simulink model "main_SIM_MMP_IIR"  (R2024a)
settings: Solver=VariableStepAuto  StartTime=0.0  StopTime=Tsim  FixedStep=simStepSize  RelTol=1e-3
undefined symbols (not defined in the file): A_amp, B_para, f_d, ForceDist, L_t, p_off, Ps_sys, Pz_sys, Qcvx_FIR, Qcvx_IIR, SensorNoise, Ts, Tu, w_k, w_k_IIR
libraries: cstblocks x4
settings Model: Creator=tomli  LastModifiedBy=tpjch
settings RTWCC: GPUComputeCapability=3.5

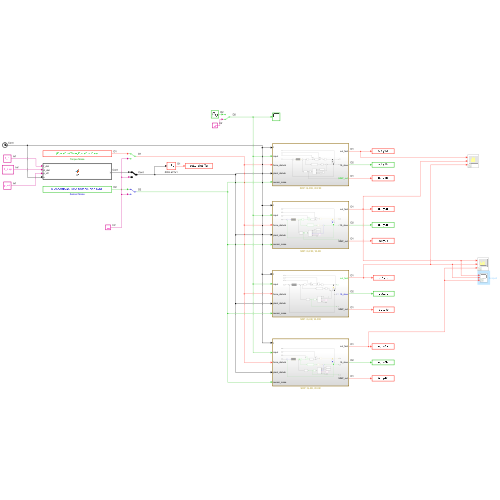
[thumbnail: Simulink's stored preview of the top-level diagram]
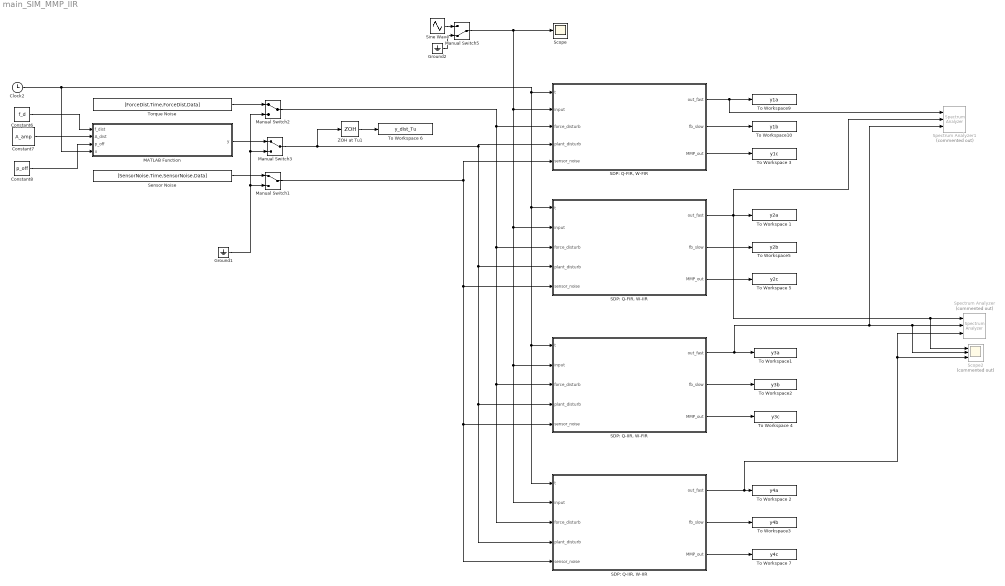
== system main_SIM_MMP_IIR ==
  Clock2 : Clock
  Constant6 : Constant  Value=f_d
  Constant7 : Constant  Value=A_amp
  Constant8 : Constant  Value=p_off
  Ground1 : Ground
  Ground2 : Ground
  MATLAB Function : MATLAB Function  TreatAsAtomicUnit=on
  Manual Switch1 : ManualSwitch
  Manual Switch2 : ManualSwitch
  Manual Switch3 : ManualSwitch
  Manual Switch5 : ManualSwitch  CurrentSetting=0
  "SDP: Q-FIR, W-FIR" : Subsystem
  "SDP: Q-FIR, W-IIR" : Subsystem
  "SDP: Q-IIR, W-FIR" : Subsystem
  "SDP: Q-IIR, W-IIR" : Subsystem
  Scope : Scope
  Scope2 : Scope  Commented=on  NumInputPorts=3
  Sensor Noise : FromWorkspace  VariableName=[SensorNoise.Time,SensorNoise.Data]  SampleTime=SensorNoise.Ts  Interpolate=off  ZeroCross=off  OutputAfterFinalValue=Setting to zero
  Sine Wave : Sin  SampleTime=Ts
  Spectrum Analyzer : SpectrumAnalyzer  Commented=on  NumInputPorts=3  WindowPosition=[1.000000,49.000000,1536.000000,888.000000,]  ScopeFrameLocation=window  Span=5280  StartFrequency=-2640  StopFrequency=2640  YLimits=[-62.09679226,16.22908912]  ShowLegend=on
  Spectrum Analyzer1 : SpectrumAnalyzer  Commented=on  NumInputPorts=3  WindowPosition=[1.000000,49.000000,1536.000000,888.000000,]  ScopeFrameLocation=window  Span=5280  StartFrequency=-2640  StopFrequency=2640  YLimits=[-59.07736824,14.75660534]  ShowLegend=on
  To Workspace 1 : ToWorkspace  VariableName=y2a  SaveFormat=Structure With Time  SampleTime=Tu
      settings: MaxDataPoints=Inf
  To Workspace 2 : ToWorkspace  VariableName=y4a  SaveFormat=Structure With Time  SampleTime=Tu
      settings: MaxDataPoints=Inf
  To Workspace 3 : ToWorkspace  VariableName=y1c  SaveFormat=Structure With Time  SampleTime=Tu
      settings: MaxDataPoints=Inf
  To Workspace 4 : ToWorkspace  VariableName=y3c  SaveFormat=Structure With Time  SampleTime=Tu
      settings: MaxDataPoints=Inf
  To Workspace 5 : ToWorkspace  VariableName=y2c  SaveFormat=Structure With Time  SampleTime=Tu
      settings: MaxDataPoints=Inf
  To Workspace 6 : ToWorkspace  VariableName=y_dist_Tu  SaveFormat=Structure With Time  SampleTime=Tu
      settings: MaxDataPoints=Inf
  To Workspace 7 : ToWorkspace  VariableName=y4c  SaveFormat=Structure With Time  SampleTime=Tu
      settings: MaxDataPoints=Inf
  To Workspace1 : ToWorkspace  VariableName=y3a  SaveFormat=Structure With Time  SampleTime=-1
  To Workspace10 : ToWorkspace  VariableName=y1b  SaveFormat=Structure With Time  SampleTime=-1
  To Workspace2 : ToWorkspace  VariableName=y3b  SaveFormat=Structure With Time  SampleTime=-1
  To Workspace3 : ToWorkspace  VariableName=y4b  SaveFormat=Structure With Time  SampleTime=Ts
  To Workspace5 : ToWorkspace  VariableName=y2b  SaveFormat=Structure With Time  SampleTime=Ts
  To Workspace9 : ToWorkspace  VariableName=y1a  SaveFormat=Structure With Time  SampleTime=-1
  Torque Noise : FromWorkspace  VariableName=[ForceDist.Time,ForceDist.Data]  SampleTime=ForceDist.Ts  Interpolate=off  ZeroCross=off  OutputAfterFinalValue=Setting to zero
  ZOH at Tu1 : ZeroOrderHold  SampleTime=Tu
  wires:
  Torque Noise/1 -> Manual Switch2/1
  Ground1/1 -> Manual Switch2/2, Manual Switch3/2, Manual Switch1/2
  Constant8/1 -> MATLAB Function/3(p_off)
  Constant7/1 -> MATLAB Function/2(A_dist)
  Constant6/1 -> MATLAB Function/1(f_dist)
  Sensor Noise/1 -> Manual Switch1/1
  MATLAB Function/1(y) -> Manual Switch3/1
  "SDP: Q-FIR, W-IIR"/3(MMP_out) -> To Workspace 5/1
  "SDP: Q-FIR, W-FIR"/1(out_fast) -> Spectrum Analyzer1/1, To Workspace9/1
  Sine Wave/1 -> Manual Switch5/1
  Ground2/1 -> Manual Switch5/2
  "SDP: Q-FIR, W-FIR"/2(fb_slow) -> To Workspace10/1
  "SDP: Q-FIR, W-IIR"/2(fb_slow) -> To Workspace5/1
  "SDP: Q-FIR, W-FIR"/3(MMP_out) -> To Workspace 3/1
  ZOH at Tu1/1 -> To Workspace 6/1
  "SDP: Q-IIR, W-FIR"/2(fb_slow) -> To Workspace2/1
  "SDP: Q-IIR, W-FIR"/3(MMP_out) -> To Workspace 4/1
  "SDP: Q-IIR, W-IIR"/2(fb_slow) -> To Workspace3/1
  "SDP: Q-IIR, W-FIR"/1(out_fast) -> Spectrum Analyzer1/3, Scope2/2, Spectrum Analyzer/2, To Workspace1/1
  Manual Switch5/1 -> "SDP: Q-IIR, W-IIR"/2(input), "SDP: Q-IIR, W-FIR"/2(input), "SDP: Q-FIR, W-IIR"/2(input), "SDP: Q-FIR, W-FIR"/2(input), Scope/1
  Manual Switch1/1 -> "SDP: Q-FIR, W-FIR"/5(sensor_noise), "SDP: Q-IIR, W-IIR"/5(sensor_noise), "SDP: Q-IIR, W-FIR"/5(sensor_noise), "SDP: Q-FIR, W-IIR"/5(sensor_noise)
  Manual Switch2/1 -> "SDP: Q-IIR, W-IIR"/3(force_disturb), "SDP: Q-IIR, W-FIR"/3(force_disturb), "SDP: Q-FIR, W-IIR"/3(force_disturb), "SDP: Q-FIR, W-FIR"/3(force_disturb)
  Clock2/1 -> "SDP: Q-IIR, W-IIR"/1(t), "SDP: Q-IIR, W-FIR"/1(t), "SDP: Q-FIR, W-IIR"/1(t), "SDP: Q-FIR, W-FIR"/1(t), MATLAB Function/4(u)
  Manual Switch3/1 -> ZOH at Tu1/1, "SDP: Q-IIR, W-IIR"/4(plant_disturb), "SDP: Q-IIR, W-FIR"/4(plant_disturb), "SDP: Q-FIR, W-IIR"/4(plant_disturb), "SDP: Q-FIR, W-FIR"/4(plant_disturb)
  "SDP: Q-IIR, W-IIR"/3(MMP_out) -> To Workspace 7/1
  "SDP: Q-IIR, W-IIR"/1(out_fast) -> Scope2/3, Spectrum Analyzer/3, To Workspace 2/1
  "SDP: Q-FIR, W-IIR"/1(out_fast) -> Spectrum Analyzer1/2, Scope2/1, Spectrum Analyzer/1, To Workspace 1/1

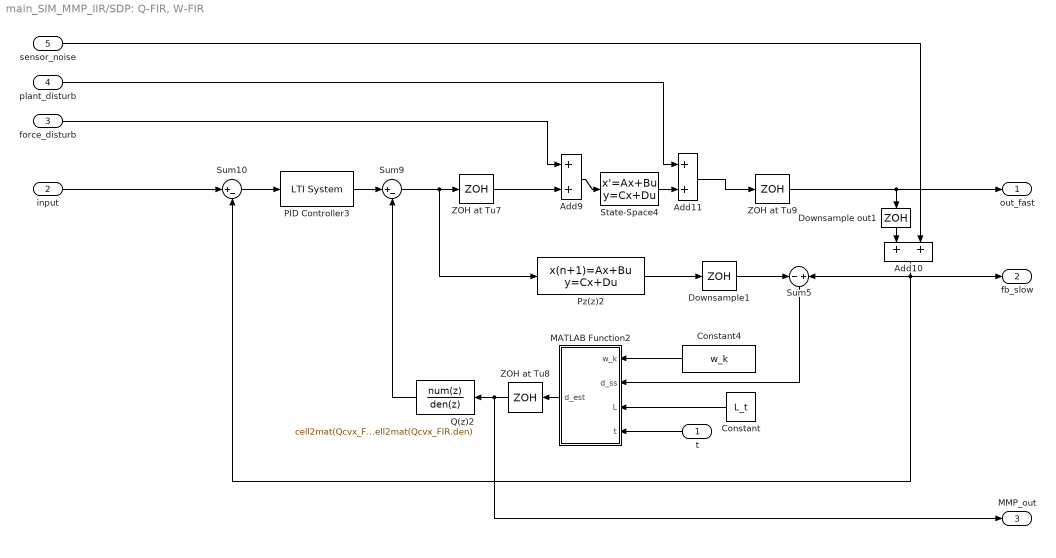
== system main_SIM_MMP_IIR/SDP: Q-FIR, W-FIR ==
  t : Inport
  input : Inport  Port=2
  force_disturb : Inport  Port=3
  plant_disturb : Inport  Port=4
  sensor_noise : Inport  Port=5
  Add10 : Sum
  Add11 : Sum
  Add9 : Sum
  Constant : Constant  Value=L_t
  Constant4 : Constant  Value=w_k
  Downsample out1 : ZeroOrderHold  SampleTime=Ts
  Downsample1 : ZeroOrderHold  SampleTime=Ts
  MATLAB Function2 : MATLAB Function  TreatAsAtomicUnit=on  SystemSampleTime=Tu
  PID Controller3 : cstblocks/LTI System  sys=Cz  IC=[]  PadeOrder=0
  Pz(z)2 : DiscreteStateSpace  A=Pz_sys.A  B=Pz_sys.B  C=Pz_sys.C  D=Pz_sys.D  SampleTime=Tu
  Q(z)2 : DiscreteTransferFcn  Numerator=cell2mat(Qcvx_FIR.num)  Denominator=cell2mat(Qcvx_FIR.den)  SampleTime=Tu
  State-Space4 : StateSpace  A=Ps_sys.A  B=Ps_sys.B  C=Ps_sys.C  D=Ps_sys.D  InitialCondition=0
  Sum10 : Sum  Inputs=|+-
  Sum5 : Sum  Inputs=-|+
  Sum9 : Sum  Inputs=|+-
  ZOH at Tu7 : ZeroOrderHold  SampleTime=Tu
  ZOH at Tu8 : ZeroOrderHold  SampleTime=Tu
  ZOH at Tu9 : ZeroOrderHold  SampleTime=Tu
  out_fast : Outport
  fb_slow : Outport  Port=2
  MMP_out : Outport  Port=3
  wires:
  ZOH at Tu9/1 -> Downsample out1/1, out_fast/1
  Sum9/1 -> Pz(z)2/1, ZOH at Tu7/1
  State-Space4/1 -> Add11/2
  Constant4/1 -> MATLAB Function2/1(w_k)
  Add10/1 -> Sum5/2, Sum10/2, fb_slow/1
  MATLAB Function2/1(d_est) -> ZOH at Tu8/1
  Add11/1 -> ZOH at Tu9/1
  force_disturb/1 -> Add9/1
  input/1 -> Sum10/1
  Pz(z)2/1 -> Downsample1/1
  ZOH at Tu8/1 -> MMP_out/1, Q(z)2/1
  Sum10/1 -> PID Controller3/1
  Add9/1 -> State-Space4/1
  Q(z)2/1 -> Sum9/2
  ZOH at Tu7/1 -> Add9/2
  Downsample1/1 -> Sum5/1
  Constant/1 -> MATLAB Function2/3(L)
  plant_disturb/1 -> Add11/1
  t/1 -> MATLAB Function2/4(t)
  sensor_noise/1 -> Add10/2
  Downsample out1/1 -> Add10/1
  Sum5/1 -> MATLAB Function2/2(d_ss)
  PID Controller3/1 -> Sum9/1

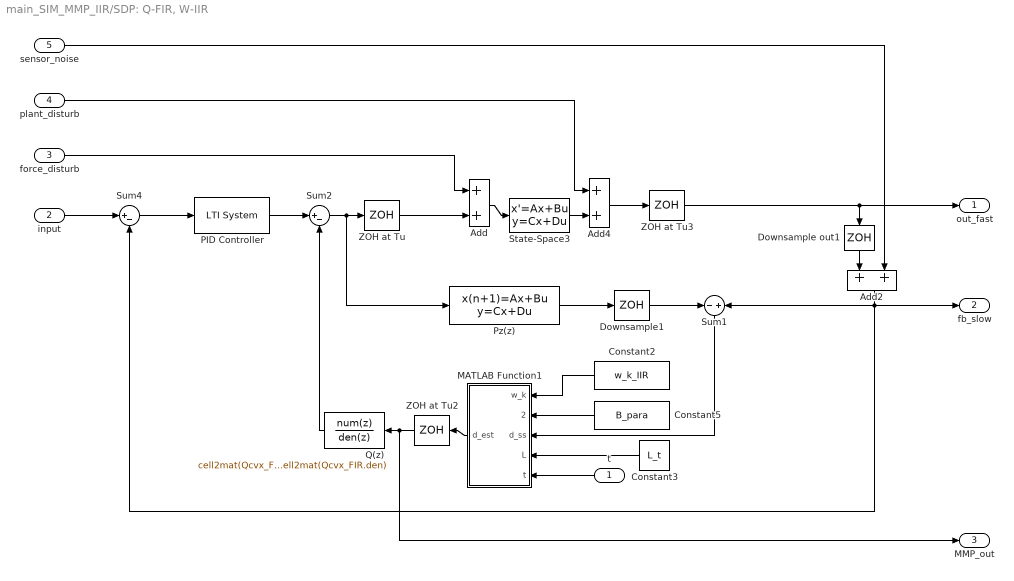
== system main_SIM_MMP_IIR/SDP: Q-FIR, W-IIR ==
  t : Inport
  input : Inport  Port=2
  force_disturb : Inport  Port=3
  plant_disturb : Inport  Port=4
  sensor_noise : Inport  Port=5
  Add : Sum
  Add2 : Sum
  Add4 : Sum
  Constant2 : Constant  Value=w_k_IIR
  Constant3 : Constant  Value=L_t
  Constant5 : Constant  Value=B_para
  Downsample out1 : ZeroOrderHold  SampleTime=Ts
  Downsample1 : ZeroOrderHold  SampleTime=Ts
  MATLAB Function1 : MATLAB Function  TreatAsAtomicUnit=on  SystemSampleTime=Tu
  PID Controller : cstblocks/LTI System  sys=Cz  IC=[]  PadeOrder=0
  Pz(z) : DiscreteStateSpace  A=Pz_sys.A  B=Pz_sys.B  C=Pz_sys.C  D=Pz_sys.D  SampleTime=Tu
  Q(z) : DiscreteTransferFcn  Numerator=cell2mat(Qcvx_FIR.num)  Denominator=cell2mat(Qcvx_FIR.den)  SampleTime=Tu
  State-Space3 : StateSpace  A=Ps_sys.A  B=Ps_sys.B  C=Ps_sys.C  D=Ps_sys.D  InitialCondition=0
  Sum1 : Sum  Inputs=-|+
  Sum2 : Sum  Inputs=|+-
  Sum4 : Sum  Inputs=|+-
  ZOH at Tu : ZeroOrderHold  SampleTime=Tu
  ZOH at Tu2 : ZeroOrderHold  SampleTime=Tu
  ZOH at Tu3 : ZeroOrderHold  SampleTime=Tu
  out_fast : Outport
  fb_slow : Outport  Port=2
  MMP_out : Outport  Port=3
  wires:
  Pz(z)/1 -> Downsample1/1
  ZOH at Tu/1 -> Add/2
  Add2/1 -> Sum1/2, Sum4/2, fb_slow/1
  Sum4/1 -> PID Controller/1
  State-Space3/1 -> Add4/2
  Downsample1/1 -> Sum1/1
  ZOH at Tu3/1 -> Downsample out1/1, out_fast/1
  Add4/1 -> ZOH at Tu3/1
  ZOH at Tu2/1 -> Q(z)/1, MMP_out/1
  Add/1 -> State-Space3/1
  Sum2/1 -> Pz(z)/1, ZOH at Tu/1
  Q(z)/1 -> Sum2/2
  force_disturb/1 -> Add/1
  plant_disturb/1 -> Add4/1
  sensor_noise/1 -> Add2/2
  input/1 -> Sum4/1
  Downsample out1/1 -> Add2/1
  Constant5/1 -> MATLAB Function1/2(B_para)
  Constant2/1 -> MATLAB Function1/1(w_k)
  MATLAB Function1/1(d_est) -> ZOH at Tu2/1
  Sum1/1 -> MATLAB Function1/3(d_ss)
  Constant3/1 -> MATLAB Function1/4(L)
  t/1 -> MATLAB Function1/5(t)
  PID Controller/1 -> Sum2/1

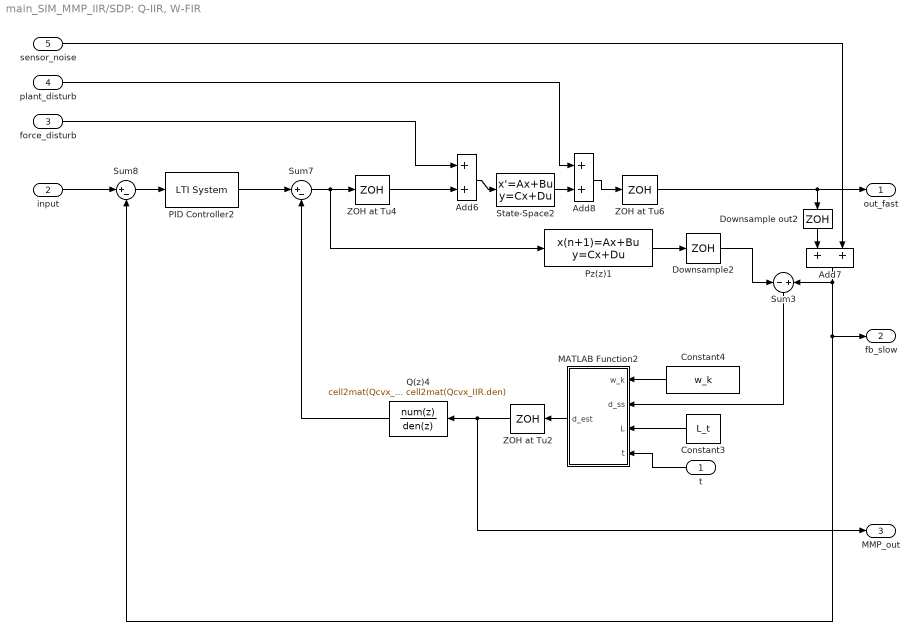
== system main_SIM_MMP_IIR/SDP: Q-IIR, W-FIR ==
  t : Inport
  input : Inport  Port=2
  force_disturb : Inport  Port=3
  plant_disturb : Inport  Port=4
  sensor_noise : Inport  Port=5
  Add6 : Sum
  Add7 : Sum
  Add8 : Sum
  Constant3 : Constant  Value=L_t
  Constant4 : Constant  Value=w_k
  Downsample out2 : ZeroOrderHold  SampleTime=Ts
  Downsample2 : ZeroOrderHold  SampleTime=Ts
  MATLAB Function2 : MATLAB Function  TreatAsAtomicUnit=on  SystemSampleTime=Tu
  PID Controller2 : cstblocks/LTI System  sys=Cz  IC=[]  PadeOrder=0
  Pz(z)1 : DiscreteStateSpace  A=Pz_sys.A  B=Pz_sys.B  C=Pz_sys.C  D=Pz_sys.D  SampleTime=Tu
  Q(z)4 : DiscreteTransferFcn  Numerator=cell2mat(Qcvx_IIR.num)  Denominator=cell2mat(Qcvx_IIR.den)
  State-Space2 : StateSpace  A=Ps_sys.A  B=Ps_sys.B  C=Ps_sys.C  D=Ps_sys.D  InitialCondition=0
  Sum3 : Sum  Inputs=-|+
  Sum7 : Sum  Inputs=|+-
  Sum8 : Sum  Inputs=|+-
  ZOH at Tu2 : ZeroOrderHold  SampleTime=Tu
  ZOH at Tu4 : ZeroOrderHold  SampleTime=Tu
  ZOH at Tu6 : ZeroOrderHold  SampleTime=Tu
  out_fast : Outport
  fb_slow : Outport  Port=2
  MMP_out : Outport  Port=3
  wires:
  Downsample2/1 -> Sum3/1
  Add8/1 -> ZOH at Tu6/1
  ZOH at Tu6/1 -> out_fast/1, Downsample out2/1
  ZOH at Tu4/1 -> Add6/2
  Add7/1 -> fb_slow/1, Sum8/2, Sum3/2
  input/1 -> Sum8/1
  sensor_noise/1 -> Add7/2
  Add6/1 -> State-Space2/1
  Sum8/1 -> PID Controller2/1
  State-Space2/1 -> Add8/2
  Sum7/1 -> Pz(z)1/1, ZOH at Tu4/1
  Pz(z)1/1 -> Downsample2/1
  plant_disturb/1 -> Add8/1
  force_disturb/1 -> Add6/1
  Downsample out2/1 -> Add7/1
  PID Controller2/1 -> Sum7/1
  Q(z)4/1 -> Sum7/2
  Constant3/1 -> MATLAB Function2/3(L)
  MATLAB Function2/1(d_est) -> ZOH at Tu2/1
  t/1 -> MATLAB Function2/4(t)
  Sum3/1 -> MATLAB Function2/2(d_ss)
  ZOH at Tu2/1 -> MMP_out/1, Q(z)4/1
  Constant4/1 -> MATLAB Function2/1(w_k)

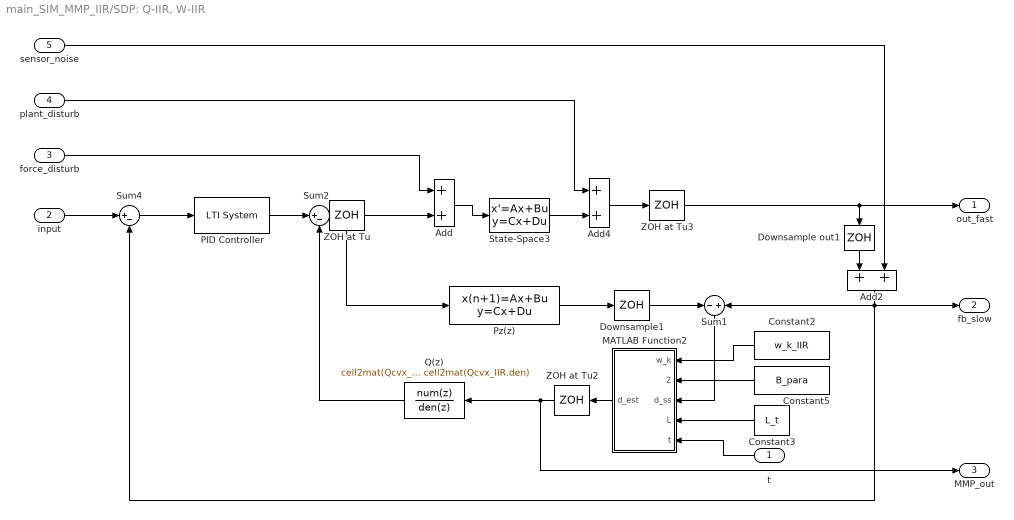
== system main_SIM_MMP_IIR/SDP: Q-IIR, W-IIR ==
  t : Inport
  input : Inport  Port=2
  force_disturb : Inport  Port=3
  plant_disturb : Inport  Port=4
  sensor_noise : Inport  Port=5
  Add : Sum
  Add2 : Sum
  Add4 : Sum
  Constant2 : Constant  Value=w_k_IIR
  Constant3 : Constant  Value=L_t
  Constant5 : Constant  Value=B_para
  Downsample out1 : ZeroOrderHold  SampleTime=Ts
  Downsample1 : ZeroOrderHold  SampleTime=Ts
  MATLAB Function2 : MATLAB Function  TreatAsAtomicUnit=on  SystemSampleTime=Tu
  PID Controller : cstblocks/LTI System  sys=Cz  IC=[]  PadeOrder=0
  Pz(z) : DiscreteStateSpace  A=Pz_sys.A  B=Pz_sys.B  C=Pz_sys.C  D=Pz_sys.D  SampleTime=Tu
  Q(z) : DiscreteTransferFcn  Numerator=cell2mat(Qcvx_IIR.num)  Denominator=cell2mat(Qcvx_IIR.den)  SampleTime=Tu
  State-Space3 : StateSpace  A=Ps_sys.A  B=Ps_sys.B  C=Ps_sys.C  D=Ps_sys.D  InitialCondition=0
  Sum1 : Sum  Inputs=-|+
  Sum2 : Sum  Inputs=|+-
  Sum4 : Sum  Inputs=|+-
  ZOH at Tu : ZeroOrderHold  SampleTime=Tu
  ZOH at Tu2 : ZeroOrderHold  SampleTime=Tu
  ZOH at Tu3 : ZeroOrderHold  SampleTime=Tu
  out_fast : Outport
  fb_slow : Outport  Port=2
  MMP_out : Outport  Port=3
  wires:
  ZOH at Tu/1 -> Add/2
  Add2/1 -> Sum1/2, Sum4/2, fb_slow/1
  Sum4/1 -> PID Controller/1
  State-Space3/1 -> Add4/2
  ZOH at Tu3/1 -> Downsample out1/1, out_fast/1
  Add4/1 -> ZOH at Tu3/1
  Add/1 -> State-Space3/1
  Sum2/1 -> Pz(z)/1, ZOH at Tu/1
  Q(z)/1 -> Sum2/2
  force_disturb/1 -> Add/1
  plant_disturb/1 -> Add4/1
  sensor_noise/1 -> Add2/2
  input/1 -> Sum4/1
  Downsample out1/1 -> Add2/1
  Constant5/1 -> MATLAB Function2/2(B_para)
  Constant2/1 -> MATLAB Function2/1(w_k)
  MATLAB Function2/1(d_est) -> ZOH at Tu2/1
  Sum1/1 -> MATLAB Function2/3(d_ss)
  Constant3/1 -> MATLAB Function2/4(L)
  t/1 -> MATLAB Function2/5(t)
  Downsample1/1 -> Sum1/1
  Pz(z)/1 -> Downsample1/1
  ZOH at Tu2/1 -> Q(z)/1, MMP_out/1
  PID Controller/1 -> Sum2/1

== matlab function main_SIM_MMP_IIR/SDP: Q-IIR, W-FIR/MATLAB Function2 ==
  settings: updateMethod=DISCRETE
  data: w_k input; d_ss input; L input; t input; d_est output
% FIR siganl reconstruction
function d_est = fcn(w_k,d_ss,L,t)
persistent phi n_fs n_ss; % keeps data of variables
n_w = height(w_k); % n_w = 2m elements (index starts at 0,1,...,2m-1)

% assigning initial values
if isempty(phi)
    phi = zeros(1,n_w);
end
if isempty(n_fs)
    n_fs = 0;
end
if isempty(n_ss)
    n_ss = 0;
end

% starts first loop with n_fs = 1 and n_ss = 1
% in MATLAB, d_ss[n_ss] = d_fs[(n_ss-1)*L+1] % for n_ss = 1, ...
% counter for loops performed
n_fs = n_fs+1; % (# of fast samples)
if mod((n_fs-1),L)==0 % update number of slow samples
    n_ss = n_ss + 1; % number of slow samples
end
k = n_fs - (n_ss-1)*L-1; % find the kth intersample point (k = 1,...,L-1)

%% case 1: n_sl < 2*m (not enough data points for FIR)
% case 1 will update phi until there is 2*m slow measured data points
% phi[n] = d_sl[n], phi(1,2m) used to temporarily store the last 2*m ...
% ... measured data points
% 1a: n_sl < 2*m and k=0 means slow and fast measurements match ...
% ... d_sl [n_sl] = d[(n_sl-1)L+1].
% need to update the new set of data points needed to start reconstruction
if (n_ss<n_w) && (k==0)
    for i = 1:(n_w-1)
    phi(n_w-i+1) = phi(n_w-i); % shifts signal data phi(1) -> phi(2)
    end
    phi(1) = d_ss; % current measured data point
    d_est = d_ss; % set d_est = d_ss since the slow and fast align
% when k ~= 0, this is the intersample point, but there is not enough ...
% ... data points, keep this off
elseif (n_ss<n_w) && k~=0 % intersample point estimation
    d_est = 0;
%% case 2: n_sl >= 2m (enough data points for FIR)
% enough data points exist for FIR signal reconstruction
elseif (n_ss>=n_w) && k==0
    for i = 1:(n_w-1)
    phi(n_w-i+1) = phi(n_w-i);
    end
    phi(1) = d_ss;
    d_est = d_ss;
else % final case: n_ss >= n_w && k~=0
    d_est = phi*w_k(:,k); % signal reconstruction step
end

== matlab function main_SIM_MMP_IIR/MATLAB Function ==
  data: f_dist input; A_dist input; p_off input; u input; y output
function y = fcn(f_dist,A_dist,p_off,u)
y = zeros(1,length(u));
for i = 1:length(f_dist)
y = y + A_dist(i)*sin(2*pi*f_dist(i)*u+p_off(i));
end

== matlab function main_SIM_MMP_IIR/SDP: Q-FIR, W-FIR/MATLAB Function2 ==
  settings: updateMethod=DISCRETE
  data: w_k input; d_ss input; L input; t input; d_est output
% FIR siganl reconstruction
function d_est = fcn(w_k,d_ss,L,t)
persistent phi n_fs n_ss; % keeps data of variables
n_w = height(w_k); % n_w = 2m elements (index starts at 0,1,...,2m-1)

% assigning initial values
if isempty(phi)
    phi = zeros(1,n_w);
end
if isempty(n_fs)
    n_fs = 0;
end
if isempty(n_ss)
    n_ss = 0;
end

% starts first loop with n_fs = 1 and n_ss = 1
% in MATLAB, d_ss[n_ss] = d_fs[(n_ss-1)*L+1] % for n_ss = 1, ...
% counter for loops performed
n_fs = n_fs+1; % (# of fast samples)
if mod((n_fs-1),L)==0 % update number of slow samples
    n_ss = n_ss + 1; % number of slow samples
end
k = n_fs - (n_ss-1)*L-1; % find the kth intersample point (k = 1,...,L-1)

%% case 1: n_sl < 2*m (not enough data points for FIR)
% case 1 will update phi until there is 2*m slow measured data points
% phi[n] = d_sl[n], phi(1,2m) used to temporarily store the last 2*m ...
% ... measured data points
% 1a: n_sl < 2*m and k=0 means slow and fast measurements match ...
% ... d_sl [n_sl] = d[(n_sl-1)L+1].
% need to update the new set of data points needed to start reconstruction
if (n_ss<n_w) && (k==0)
    for i = 1:(n_w-1)
    phi(n_w-i+1) = phi(n_w-i); % shifts signal data phi(1) -> phi(2)
    end
    phi(1) = d_ss; % current measured data point
    d_est = d_ss; % set d_est = d_ss since the slow and fast align
% when k ~= 0, this is the intersample point, but there is not enough ...
% ... data points, keep this off
elseif (n_ss<n_w) && k~=0 % intersample point estimation
    d_est = 0;
%% case 2: n_sl >= 2m (enough data points for FIR)
% enough data points exist for FIR signal reconstruction
elseif (n_ss>=n_w) && k==0
    for i = 1:(n_w-1)
    phi(n_w-i+1) = phi(n_w-i);
    end
    phi(1) = d_ss;
    d_est = d_ss;
else % final case: n_ss >= n_w && k~=0
    d_est = phi*w_k(:,k); % signal reconstruction step
end

== matlab function main_SIM_MMP_IIR/SDP: Q-FIR, W-IIR/MATLAB Function1 ==
  settings: updateMethod=DISCRETE
  data: w_k input; B_para input; d_ss input; L input; t input; d_est output
% IIR signal reconstruction based on 2018 paper. Rejecting fast narrow-band
% disturbances with slow sensor feedback for quality beam steering in
% selective laser sintering (Xiao, H.; Jiang, T; Chen, X.)
function d_est = fcn(w_k, B_para, d_ss,L,t) % keeps data of variables
persistent phi n_fs n_ss d_IIR;
n_w = height(w_k); % n_w = 2m elements (index starts at 0,1,...,2m-1)

% assigning initial values
if isempty(phi)
    phi = zeros(1,n_w);
end
if isempty(n_fs)
    n_fs = 0; % fast sampling count
end
if isempty(n_ss)
    n_ss = 0; % slow sampling count
end
if isempty(d_IIR)
    d_IIR = zeros(1,0); % stored fast sampling signal
end

% starts first loop with n_fs = 1 and n_ss = 1
% in MATLAB, d_ss[n_ss] = d_fs[(n_ss-1)*L+1] % for n_ss = 1, ...
% counter for loops performed
n_fs = n_fs+1; % (# of fast samples)
if mod((n_fs-1),L)==0 % update number of slow samples
    n_ss = n_ss + 1; % number of slow samples
end
k = n_fs - (n_ss-1)*L-1; % find the kth intersample point (k = 1,...,L-1)

%% case 1: n_sl < 2*m (not enough data points for FIR)
% case 1 will update phi until there is 2*m slow measured data points
% phi[n] = d_sl[n], phi(1,2m) used to temporarily store the last 2*m ...
% ... measured data points
% 1a: n_sl < 2*m and k=0 means slow and fast measurements match ...
% ... d_sl [n_sl] = d[(n_sl-1)L+1].
% need to update the new set of data points needed to start reconstruction
if (n_ss < n_w) && (k==0)
    for i = 1:(n_w-1)
    phi(n_w-i+1) = phi(n_w-i); % shifts signal data phi(1) -> phi(2)
    end
    phi(1) = d_ss; % current measured data point
    d_est = d_ss; % set d_est = d_ss since the slow and fast align
    d_IIR(end+1) = d_est;
% when k ~= 0, this is the intersample point, but there is not enough ...
% ... data points, keep this off
% elseif (n_ss < n_w) && (k~=0) % intersample point estimation
elseif (n_ss < n_w) && (k~=0) % intersample point estimation
    d_est = 0;
    d_IIR(end+1) = d_est;
%% case 2: n_sl >= 2m (enough data points for FIR)
% enough data points exist to start FIR signal reconstruction
elseif  (n_ss >= n_w) && (n_ss < (n_w+1)) && (k==0) 
    for i = 1:(n_w-1)
    phi(n_w-i+1) = phi(n_w-i);
    end
    phi(1) = d_ss;
    d_est = d_ss;
    d_IIR(end+1) = d_ss;
elseif (n_ss >= n_w) && (n_ss < (n_w+1)) && (k~=0) % intersmaple point
    % d_est = phi*w_k(:,k);
    d_est = 0;
    d_IIR(end+1) = d_est;
%% case 3: n_sl >= 2m+1 (enough data points for IIR)
elseif (n_ss >= (n_w+1)) && k==0
    for i = 1:(n_w-1)
    phi(n_w-i+1) = phi(n_w-i);
    end
    phi(1) = d_ss;
    d_est = d_ss;
    d_IIR(end+1) = d_est;
else % n_ss>=(n_w+1) && k~=0
    d_est = phi*w_k(:,k)-...
    flip(d_IIR(((n_ss-n_w-1)*L+k+1):L:((n_ss-2)*L+k+1)))*B_para(2:end);
    d_IIR(end+1) = d_est;
end

== matlab function main_SIM_MMP_IIR/SDP: Q-IIR, W-IIR/MATLAB Function2 ==
  settings: updateMethod=DISCRETE
  data: w_k input; B_para input; d_ss input; L input; t input; d_est output
% IIR signal reconstruction based on 2018 paper. Rejecting fast narrow-band
% disturbances with slow sensor feedback for quality beam steering in
% selective laser sintering (Xiao, H.; Jiang, T; Chen, X.)
function d_est  = fcn(w_k, B_para, d_ss,L,t) % keeps data of variables
persistent phi n_fs n_ss d_IIR;
n_w = height(w_k); % n_w = 2m elements (index starts at 0,1,...,2m-1)

% assigning initial values
if isempty(phi)
    phi = zeros(1,n_w);
end
if isempty(n_fs)
    n_fs = 0; % fast sampling count
end
if isempty(n_ss)
    n_ss = 0; % slow sampling count
end
if isempty(d_IIR)
    d_IIR = zeros(1,0); % stored fast sampling signal
end

% starts first loop with n_fs = 1 and n_ss = 1
% in MATLAB, d_ss[n_ss] = d_fs[(n_ss-1)*L+1] % for n_ss = 1, ...
% counter for loops performed
n_fs = n_fs+1; % (# of fast samples)
if mod((n_fs-1),L)==0 % update number of slow samples
    n_ss = n_ss + 1; % number of slow samples
end
k = n_fs - (n_ss-1)*L-1; % find the kth intersample point (k = 1,...,L-1)
%% case 1: n_sl < 2*m (not enough data points for FIR)
% case 1 will update phi until there is 2*m slow measured data points
% phi[n] = d_sl[n], phi(1,2m) used to temporarily store the last 2*m ...
% ... measured data points
% 1a: n_sl < 2*m and k=0 means slow and fast measurements match ...
% ... d_sl [n_sl] = d[(n_sl-1)L+1].
% need to update the new set of data points needed to start reconstruction
if (n_ss < n_w) && (k==0)
    for i = 1:(n_w-1)
    phi(n_w-i+1) = phi(n_w-i); % shifts signal data phi(1) -> phi(2)
    end
    phi(1) = d_ss; % current measured data point
    d_est = d_ss; % set d_est = d_ss since the slow and fast align
    d_IIR(end+1) = d_est;
% when k ~= 0, this is the intersample point, but there is not enough ...
% ... data points, keep this off
% elseif (n_ss < n_w) && (k~=0) % intersample point estimation
elseif (n_ss < n_w) && (k~=0) % intersample point estimation
    d_est = 0;
    d_IIR(end+1) = d_est;
%% case 2: n_sl >= 2m (enough data points for FIR)
% enough data points exist to start FIR signal reconstruction
elseif  (n_ss >= n_w) && (n_ss < (n_w+1)) && (k==0) 
    for i = 1:(n_w-1)
    phi(n_w-i+1) = phi(n_w-i);
    end
    phi(1) = d_ss;
    d_est = d_ss;
    d_IIR(end+1) = d_ss;
elseif (n_ss >= n_w) && (n_ss < (n_w+1)) && (k~=0) % intersmaple point
    % d_est = phi*w_k(:,k);
    d_est = 0;
    d_IIR(end+1) = d_est;
%% case 3: n_sl >= 2m+1 (enough data points for IIR)
elseif (n_ss >= (n_w+1)) && k==0
    for i = 1:(n_w-1)
    phi(n_w-i+1) = phi(n_w-i);
    end
    phi(1) = d_ss;
    d_est = d_ss;
    d_IIR(end+1) = d_est;
else % n_ss>=(n_w+1) && k~=0
    d_est = phi*w_k(:,k)-...
    flip(d_IIR(((n_ss-n_w-1)*L+k+1):L:((n_ss-2)*L+k+1)))*B_para(2:end);
    d_IIR(end+1) = d_est;
end
